simulink model "SLIPquadwalkold"  (R2015a)
settings: Solver=ode45  StartTime=0.0  StopTime=10  MaxStep=1e-3  RelTol=1e-4  AbsTol=1e-6
values from neighbouring files (symbols this model uses):
  blic = 0    [SLIPquad_paramswalk.m]    (also in purecmaeswalk.m; test.m)
  blx0 = x(10)    [SLIPquad_paramswalk.m]    (also in purecmaeswalk.m; test.m)
  bric = 1    [SLIPquad_paramswalk.m]    (also in purecmaeswalk.m; test.m)
  brx0 = 0    [SLIPquad_paramswalk.m]    (also in purecmaeswalk.m; test.m)
  flic = 0    [SLIPquad_paramswalk.m]    (also in purecmaeswalk.m; test.m)
  flx0 = x(9)    [SLIPquad_paramswalk.m]    (also in purecmaeswalk.m; test.m)
  fric = 1    [SLIPquad_paramswalk.m]    (also in purecmaeswalk.m; test.m)
  frx0 = 0    [SLIPquad_paramswalk.m]    (also in purecmaeswalk.m; test.m)
  g = 9.81    [SLIPquad_params - Copy.m]    (also in SLIPquad_params.m; SLIPquad_paramswalk.m; purecmaes.m; purecmaeswalk.m)
  J = 4.58    [SLIPquad_params - Copy.m]    (also in SLIPquad_params.m; SLIPquad_paramswalk.m; purecmaes.m; purecmaeswalk.m)
  L = 0.5    [SLIPquad_params - Copy.m]    (also in SLIPquad_params.m; SLIPquad_paramswalk.m; purecmaes.m; purecmaeswalk.m)
  l0 = 1    [SLIPquad_params - Copy.m]    (also in SLIPquad_params.m; SLIPquad_paramswalk.m; purecmaes.m; purecmaeswalk.m)
  m = 80    [SLIPquad_params - Copy.m]    (also in SLIPquad_params.m; SLIPquad_paramswalk.m; purecmaes.m; purecmaeswalk.m)
libraries: simulink_extras x4, dspswit3 x1
settings Model: Creator=hgeyer  LastModifiedBy=Joe
settings DataIOCC: LimitDataPoints=off  SignalLoggingSaveFormat=ModelDataLogs
settings OptimizationCC: ExpressionDepthLimit=2147483647
settings DebuggingCC: UnderspecifiedInitializationDetection=Classic  MergeDetectMultiDrivingBlocksExec=none  SolverPrmCheckMsg=warning  FcnCallInpInsideContextMsg=EnableAllAsWarning  StateNameClashWarn=warning

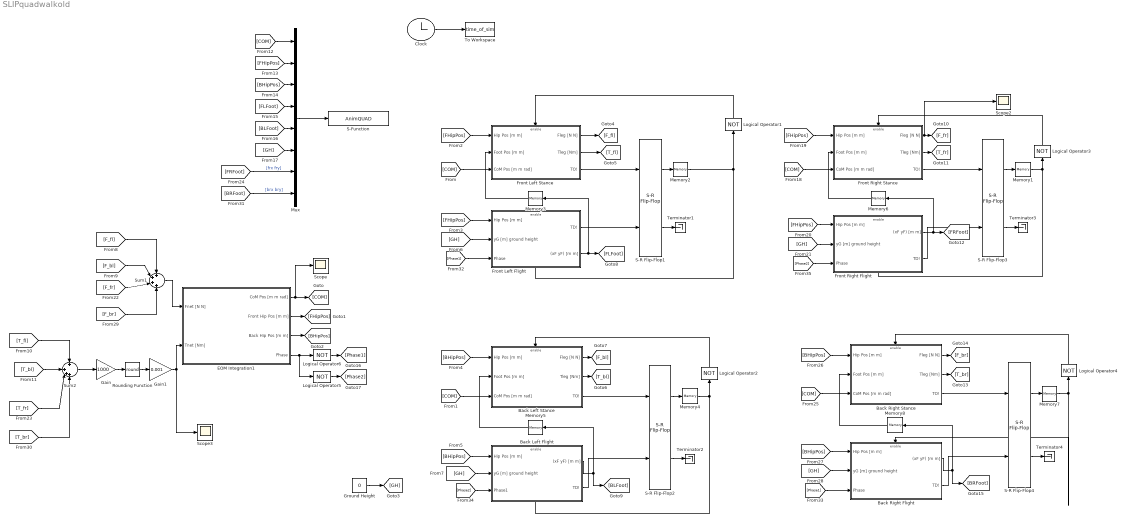
== system SLIPquadwalkold ==
  Back Left Flight : Subsystem
  Back Left Stance : Subsystem
  Back Right Flight : Subsystem
  Back Right Stance : Subsystem
  Clock : Clock
      settings: Decimation=100
  EOM Integration1 : Subsystem
  Front Left Flight : Subsystem
  Front Left Stance : Subsystem
  Front Right Flight : Subsystem
  Front Right Stance : Subsystem
  Gain : Gain  Gain=1000
  Gain1 : Gain  Gain=0.001
  Ground Height : Constant  Value=0
  Logical Operator{1..6} (6 alike) : Logic  Operator=NOT  AllPortsSameDT=off  OutDataTypeStr=boolean
  Memory1 : Memory  X0=fric
  Memory2 : Memory  X0=flic
  Memory3 : Memory  X0=[flx0 0]
  Memory4 : Memory  X0=blic
  Memory5 : Memory  X0=[blx0 0]
  Memory6 : Memory  X0=[frx0 0]
  Memory7 : Memory  X0=bric
  Memory8 : Memory  X0=[brx0 0]
  Mux : Mux  Inputs=8
  Rounding Function : Rounding  Operator=round
  S-Function : S-Function  FunctionName=AnimQUAD  Parameters=0.005  SFunctionDeploymentMode=off  EnableBusSupport=off
  S-R Flip-Flop1 : simulink_extras/Flip Flops/S-R Flip-Flop  initial_condition=flic
  S-R Flip-Flop2 : simulink_extras/Flip Flops/S-R Flip-Flop  initial_condition=blic
  S-R Flip-Flop3 : simulink_extras/Flip Flops/S-R Flip-Flop  initial_condition=fric
  S-R Flip-Flop4 : simulink_extras/Flip Flops/S-R Flip-Flop  initial_condition=bric
  Scope : Scope
      settings: TimeRange=auto  MaxDataPoints=5000  SaveToWorkspace=off  SaveName=ScopeData  YMin=-0.16878  YMax=0.96227  SampleTime=-1  DataFormat=Array
  Scope2 : Scope
      settings: TimeRange=auto  LimitDataPoints=on  MaxDataPoints=5000  SaveToWorkspace=off  SaveName=ScopeData3  YMin=-10  YMax=10  SampleTime=-1  DataFormat=Array
  Scope3 : Scope
      settings: TimeRange=auto  MaxDataPoints=5000  SaveToWorkspace=off  SaveName=ScopeData4  YMin=-0.05618  YMax=0.0173  SampleTime=-1  DataFormat=Array
  Sum1 : Sum  Inputs=++++
  Sum2 : Sum  Inputs=+|+++
  Terminator{1..4} (4 alike) : Terminator
  To Workspace : ToWorkspace  VariableName=time_of_sim  SampleTime=-1
      settings: MaxDataPoints=1
  wires:
  Front Left Stance/3(TO!) -> S-R Flip-Flop1/1
  S-R Flip-Flop1/1 -> Memory2/1
  Front Left Flight/1(TD!) -> S-R Flip-Flop1/2
  Logical Operator1/1 -> Front Left Stance/Enable
  S-R Flip-Flop1/2 -> Terminator1/1
  Front Left Flight/2((xF yF) [m m]) -> [FLFoot], Memory3/1
  Memory3/1 -> Front Left Stance/2(Foot Pos [m m])
  Back Left Stance/3(TO!) -> S-R Flip-Flop2/1
  S-R Flip-Flop2/1 -> Memory4/1
  Back Left Flight/2(TD!) -> S-R Flip-Flop2/2
  Memory4/1 -> Back Left Flight/Enable, Logical Operator2/1
  Logical Operator2/1 -> Back Left Stance/Enable
  S-R Flip-Flop2/2 -> Terminator2/1
  [GH] -> Back Left Flight/2(yG [m] ground height)
  Back Left Flight/1((xF yF) [m m]) -> [BLFoot], Memory5/1
  Memory5/1 -> Back Left Stance/2(Foot Pos [m m])
  Ground Height/1 -> [GH]
  [GH] -> Front Left Flight/2(yG [m] ground height)
  Front Left Stance/1(Fleg [N N]) -> [F_fl]
  Front Left Stance/2(Tleg [Nm]) -> [T_fl]
  Back Left Stance/1(Fleg [N N]) -> [F_bl]
  Back Left Stance/2(Tleg [Nm]) -> [T_bl]
  [F_fl] -> Sum1/1
  [F_bl] -> Sum1/2
  [T_fl] -> Sum2/1
  [T_bl] -> Sum2/2
  Sum1/1 -> EOM Integration1/1(Fnet [N N])
  EOM Integration1/1(CoM Pos [m m rad]) -> Scope/1, [COM]
  EOM Integration1/2(Front Hip Pos [m m]) -> [FHipPos]
  EOM Integration1/3(Back Hip Pos [m m]) -> [BHipPos]
  [FHipPos] -> Front Left Stance/1(Hip Pos [m m])
  [FHipPos] -> Front Left Flight/1(Hip Pos [m m])
  [BHipPos] -> Back Left Stance/1(Hip Pos [m m])
  [BHipPos] -> Back Left Flight/1(Hip Pos [m m])
  [COM] -> Front Left Stance/3(CoM Pos [m m rad])
  [COM] -> Back Left Stance/3(CoM Pos [m m rad])
  Sum2/1 -> Gain/1
  Gain1/1 -> Scope3/1, EOM Integration1/2(Tnet [Nm])
  Gain/1 -> Rounding Function/1
  Rounding Function/1 -> Gain1/1
  Mux/1 -> S-Function/1
  [COM] -> Mux/1
  [FHipPos] -> Mux/2
  [BHipPos] -> Mux/3
  [FLFoot] -> Mux/4
  [BLFoot] -> Mux/5
  [GH] -> Mux/6
  [FRFoot] -> Mux/7  "[frx fry]"
  [BRFoot] -> Mux/8  "[brx bry]"
  Front Right Stance/3(TO!) -> S-R Flip-Flop3/1
  S-R Flip-Flop3/1 -> Memory1/1
  Front Right Flight/2(TD!) -> S-R Flip-Flop3/2
  Memory1/1 -> Front Right Flight/Enable, Logical Operator3/1
  Logical Operator3/1 -> Front Right Stance/Enable
  S-R Flip-Flop3/2 -> Terminator3/1
  Front Right Flight/1((xF yF) [m m]) -> Memory6/1, [FRFoot]
  Memory6/1 -> Front Right Stance/2(Foot Pos [m m])
  [GH] -> Front Right Flight/2(yG [m] ground height)
  Front Right Stance/1(Fleg [N N]) -> Scope2/1, [F_fr]
  Front Right Stance/2(Tleg [Nm]) -> [T_fr]
  [FHipPos] -> Front Right Stance/1(Hip Pos [m m])
  [FHipPos] -> Front Right Flight/1(Hip Pos [m m])
  [COM] -> Front Right Stance/3(CoM Pos [m m rad])
  [F_fr] -> Sum1/3
  [T_fr] -> Sum2/3
  Back Right Stance/3(TO!) -> S-R Flip-Flop4/1
  S-R Flip-Flop4/1 -> Memory7/1
  Back Right Flight/2(TD!) -> S-R Flip-Flop4/2
  Memory7/1 -> Back Right Flight/Enable, Logical Operator4/1
  Logical Operator4/1 -> Back Right Stance/Enable
  S-R Flip-Flop4/2 -> Terminator4/1
  [GH] -> Back Right Flight/2(yG [m] ground height)
  Back Right Flight/1((xF yF) [m m]) -> [BRFoot], Memory8/1
  Memory8/1 -> Back Right Stance/2(Foot Pos [m m])
  Back Right Stance/1(Fleg [N N]) -> [F_br]
  Back Right Stance/2(Tleg [Nm]) -> [T_br]
  [BHipPos] -> Back Right Stance/1(Hip Pos [m m])
  [BHipPos] -> Back Right Flight/1(Hip Pos [m m])
  [COM] -> Back Right Stance/3(CoM Pos [m m rad])
  [F_br] -> Sum1/4
  [T_br] -> Sum2/4
  Clock/1 -> To Workspace/1
  EOM Integration1/4(Phase) -> Logical Operator5/1, Logical Operator6/1
  [Phase1] -> Front Left Flight/3(Phase)
  [Phase1] -> Back Right Flight/3(Phase)
  [Phase2] -> Back Left Flight/3(Phase1)
  [Phase2] -> Front Right Flight/3(Phase)
  Logical Operator5/1 -> [Phase2]
  Logical Operator6/1 -> [Phase1]
  Memory2/1 -> Front Left Flight/Enable, Logical Operator1/1

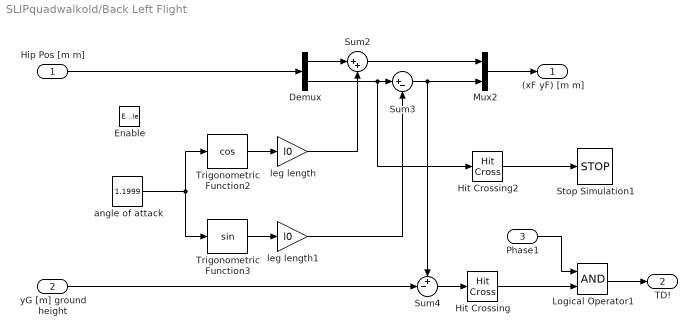
== system SLIPquadwalkold/Back Left Flight ==
  Hip Pos [m m] : Inport
  yG [m] ground height : Inport  Port=2
  Phase1 : Inport  Port=3
  Enable : EnablePort  StatesWhenEnabling=reset
  Demux : Demux  Outputs=2
  Hit Crossing : HitCross  HitCrossingDirection=falling
  Hit Crossing2 : HitCross  HitCrossingOffset=-1  HitCrossingDirection=falling
  Logical Operator1 : Logic  AllPortsSameDT=off  OutDataTypeStr=boolean
  Mux2 : Mux  Inputs=2
  Stop Simulation1 : Stop
  Sum2 : Sum  Inputs=|++
  Sum3 : Sum  Inputs=|+-
  Sum4 : Sum  Inputs=+-|
  Trigonometric Function2 : Trigonometry  Operator=cos
  Trigonometric Function3 : Trigonometry
  angle of attack : Constant  Value=1.1999
  leg length : Gain  Gain=l0
  leg length1 : Gain  Gain=l0
  (xF yF) [m m] : Outport  InitialOutput=[blx0 0]
      settings: AttributesFormatString=%<OutputWhenDisabled>
  TD! : Outport  Port=2  OutputWhenDisabled=reset  InitialOutput=0
      settings: AttributesFormatString=%<OutputWhenDisabled>
  wires:
  Demux/2 -> Hit Crossing2/1, Sum3/1
  Demux/1 -> Sum2/1
  angle of attack/1 -> Trigonometric Function3/1, Trigonometric Function2/1
  Trigonometric Function2/1 -> leg length/1
  Trigonometric Function3/1 -> leg length1/1
  Hip Pos [m m]/1 -> Demux/1
  leg length/1 -> Sum2/2
  leg length1/1 -> Sum3/2
  Sum3/1 -> Mux2/2, Sum4/1
  Sum2/1 -> Mux2/1
  Mux2/1 -> (xF yF) [m m]/1
  yG [m] ground height/1 -> Sum4/2
  Sum4/1 -> Hit Crossing/1
  Hit Crossing2/1 -> Stop Simulation1/1
  Hit Crossing/1 -> Logical Operator1/2
  Phase1/1 -> Logical Operator1/1
  Logical Operator1/1 -> TD!/1

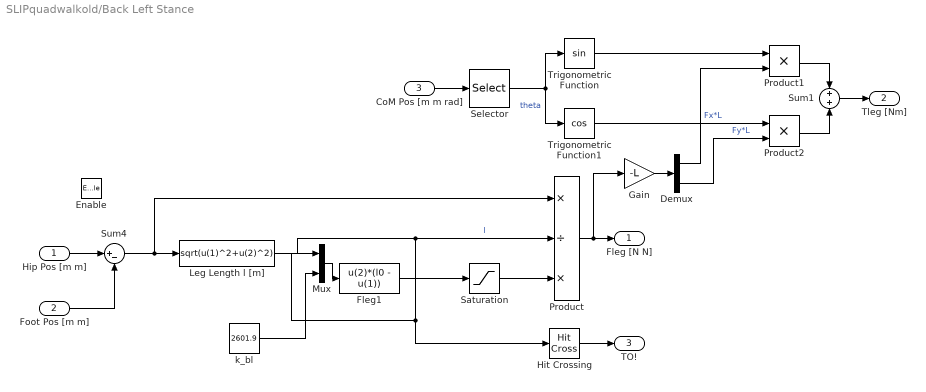
== system SLIPquadwalkold/Back Left Stance ==
  Hip Pos [m m] : Inport
  Foot Pos [m m] : Inport  Port=2
  CoM Pos [m m rad] : Inport  Port=3
  Enable : EnablePort  StatesWhenEnabling=reset
  Demux : Demux  Outputs=2
  Fleg1 : Fcn  Expr=u(2)*(l0 - u(1))
  Gain : Gain  Gain=-L
  Hit Crossing : HitCross  HitCrossingOffset=l0  HitCrossingDirection=rising
  Leg Length l [m] : Fcn  Expr=sqrt(u(1)^2+u(2)^2)
  Mux : Mux  Inputs=2
  Product : Product  Inputs=*/*
  Product1 : Product
  Product2 : Product
  Saturation : Saturate  UpperLimit=Inf  LowerLimit=0
  Selector : Selector  InputPortWidth=3  IndexOptions=Index vector (dialog)  Indices=[3]  OutputSizes=1
  Sum1 : Sum  Inputs=+|+
  Sum4 : Sum  Inputs=|+-
  Trigonometric Function : Trigonometry
  Trigonometric Function1 : Trigonometry  Operator=cos
  k_bl : Constant  Value=2601.9
  Fleg [N N] : Outport  OutputWhenDisabled=reset  InitialOutput=[0 0]
      settings: AttributesFormatString=%<OutputWhenDisabled>
  Tleg [Nm] : Outport  Port=2  OutputWhenDisabled=reset  InitialOutput=[0]
      settings: AttributesFormatString=%<OutputWhenDisabled>
  TO! : Outport  Port=3  OutputWhenDisabled=reset  InitialOutput=[0]
      settings: AttributesFormatString=%<OutputWhenDisabled>
  wires:
  Sum1/1 -> Tleg [Nm]/1
  Product1/1 -> Sum1/1
  Product2/1 -> Sum1/2
  Gain/1 -> Demux/1
  Demux/2 -> Product2/2  "Fy*L"
  Demux/1 -> Product1/2  "Fx*L"
  Trigonometric Function/1 -> Product1/1
  Trigonometric Function1/1 -> Product2/1
  Selector/1 -> Trigonometric Function/1, Trigonometric Function1/1  "theta"
  CoM Pos [m m rad]/1 -> Selector/1
  Foot Pos [m m]/1 -> Sum4/2
  Hip Pos [m m]/1 -> Sum4/1
  Hit Crossing/1 -> TO!/1
  Product/1 -> Fleg [N N]/1, Gain/1
  Fleg1/1 -> Saturation/1
  Leg Length l [m]/1 -> Hit Crossing/1, Mux/1, Product/2  "l"
  Sum4/1 -> Leg Length l [m]/1, Product/1
  Mux/1 -> Fleg1/1
  k_bl/1 -> Mux/2
  Saturation/1 -> Product/3

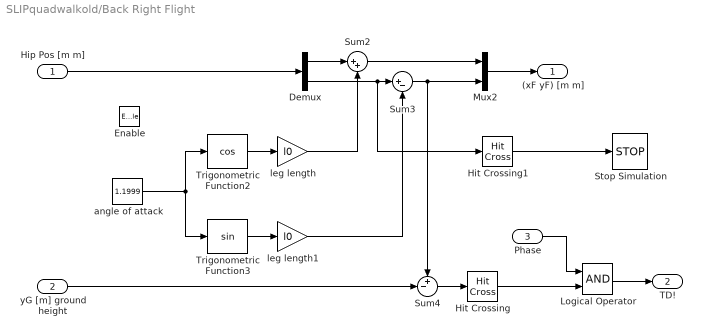
== system SLIPquadwalkold/Back Right Flight ==
  Hip Pos [m m] : Inport
  yG [m] ground height : Inport  Port=2
  Phase : Inport  Port=3
  Enable : EnablePort  StatesWhenEnabling=reset
  Demux : Demux  Outputs=2
  Hit Crossing : HitCross  HitCrossingDirection=falling
  Hit Crossing1 : HitCross  HitCrossingOffset=-1  HitCrossingDirection=falling
  Logical Operator : Logic  AllPortsSameDT=off  OutDataTypeStr=boolean
  Mux2 : Mux  Inputs=2
  Stop Simulation : Stop
  Sum2 : Sum  Inputs=|++
  Sum3 : Sum  Inputs=|+-
  Sum4 : Sum  Inputs=+-|
  Trigonometric Function2 : Trigonometry  Operator=cos
  Trigonometric Function3 : Trigonometry
  angle of attack : Constant  Value=1.1999
  leg length : Gain  Gain=l0
  leg length1 : Gain  Gain=l0
  (xF yF) [m m] : Outport  InitialOutput=[brx0 0]
      settings: AttributesFormatString=%<OutputWhenDisabled>
  TD! : Outport  Port=2  OutputWhenDisabled=reset  InitialOutput=0
      settings: AttributesFormatString=%<OutputWhenDisabled>
  wires:
  Demux/2 -> Hit Crossing1/1, Sum3/1
  Demux/1 -> Sum2/1
  angle of attack/1 -> Trigonometric Function3/1, Trigonometric Function2/1
  Trigonometric Function2/1 -> leg length/1
  Trigonometric Function3/1 -> leg length1/1
  Hip Pos [m m]/1 -> Demux/1
  leg length/1 -> Sum2/2
  leg length1/1 -> Sum3/2
  Sum3/1 -> Mux2/2, Sum4/1
  Sum2/1 -> Mux2/1
  Mux2/1 -> (xF yF) [m m]/1
  yG [m] ground height/1 -> Sum4/2
  Sum4/1 -> Hit Crossing/1
  Hit Crossing1/1 -> Stop Simulation/1
  Hit Crossing/1 -> Logical Operator/2
  Phase/1 -> Logical Operator/1
  Logical Operator/1 -> TD!/1

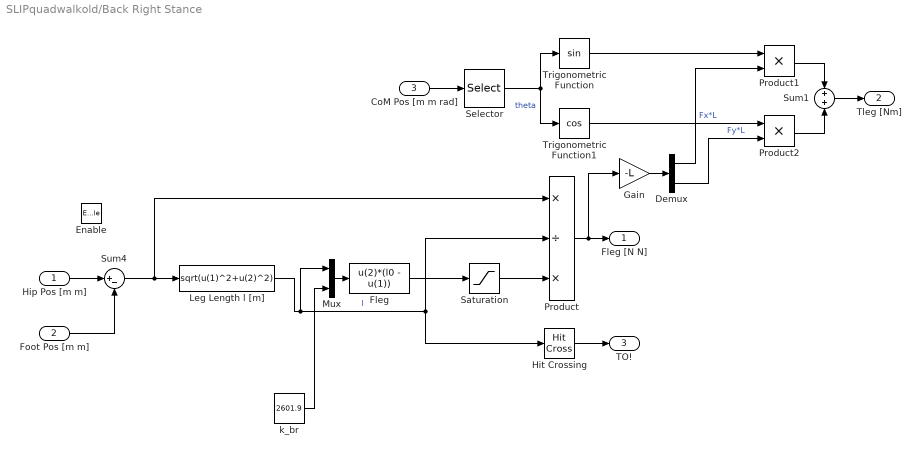
== system SLIPquadwalkold/Back Right Stance ==
  Hip Pos [m m] : Inport
  Foot Pos [m m] : Inport  Port=2
  CoM Pos [m m rad] : Inport  Port=3
  Enable : EnablePort  StatesWhenEnabling=reset
  Demux : Demux  Outputs=2
  Fleg : Fcn  Expr=u(2)*(l0 - u(1))
  Gain : Gain  Gain=-L
  Hit Crossing : HitCross  HitCrossingOffset=l0  HitCrossingDirection=rising
  Leg Length l [m] : Fcn  Expr=sqrt(u(1)^2+u(2)^2)
  Mux : Mux  Inputs=2
  Product : Product  Inputs=*/*
  Product1 : Product
  Product2 : Product
  Saturation : Saturate  UpperLimit=Inf  LowerLimit=0
  Selector : Selector  InputPortWidth=3  IndexOptions=Index vector (dialog)  Indices=[3]  OutputSizes=1
  Sum1 : Sum  Inputs=+|+
  Sum4 : Sum  Inputs=|+-
  Trigonometric Function : Trigonometry
  Trigonometric Function1 : Trigonometry  Operator=cos
  k_br : Constant  Value=2601.9
  Fleg [N N] : Outport  OutputWhenDisabled=reset  InitialOutput=[0 0]
      settings: AttributesFormatString=%<OutputWhenDisabled>
  Tleg [Nm] : Outport  Port=2  OutputWhenDisabled=reset  InitialOutput=[0]
      settings: AttributesFormatString=%<OutputWhenDisabled>
  TO! : Outport  Port=3  OutputWhenDisabled=reset  InitialOutput=[0]
      settings: AttributesFormatString=%<OutputWhenDisabled>
  wires:
  Sum1/1 -> Tleg [Nm]/1
  Product1/1 -> Sum1/1
  Product2/1 -> Sum1/2
  Gain/1 -> Demux/1
  Demux/2 -> Product2/2  "Fy*L"
  Demux/1 -> Product1/2  "Fx*L"
  Trigonometric Function/1 -> Product1/1
  Trigonometric Function1/1 -> Product2/1
  Selector/1 -> Trigonometric Function/1, Trigonometric Function1/1  "theta"
  CoM Pos [m m rad]/1 -> Selector/1
  Foot Pos [m m]/1 -> Sum4/2
  Hip Pos [m m]/1 -> Sum4/1
  Hit Crossing/1 -> TO!/1
  Product/1 -> Fleg [N N]/1, Gain/1
  Fleg/1 -> Saturation/1
  Leg Length l [m]/1 -> Hit Crossing/1, Product/2, Mux/1  "l"
  Sum4/1 -> Leg Length l [m]/1, Product/1
  Mux/1 -> Fleg/1
  k_br/1 -> Mux/2
  Saturation/1 -> Product/3

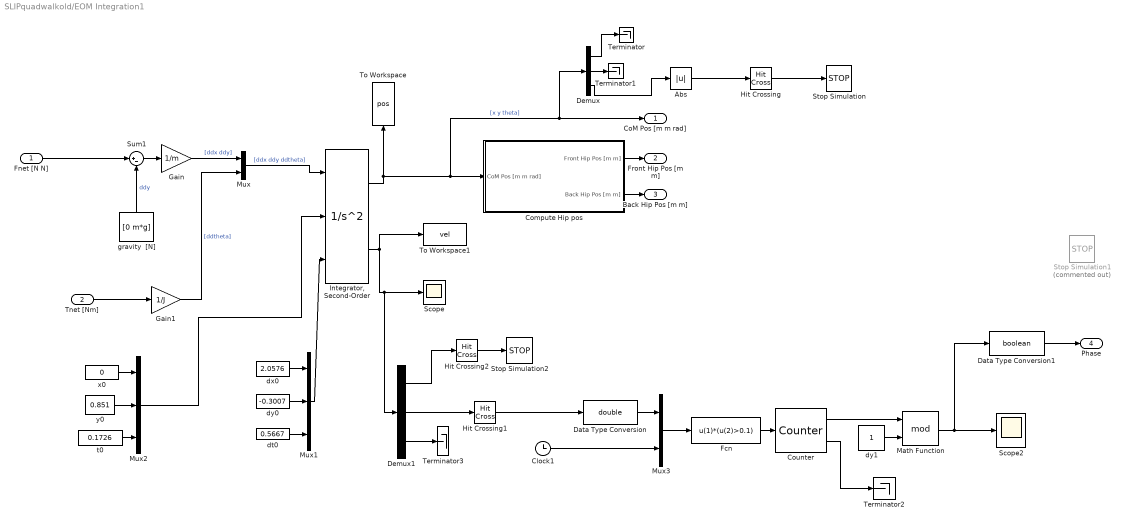
== system SLIPquadwalkold/EOM Integration1 ==
  Fnet [N N] : Inport
  Tnet [Nm] : Inport  Port=2
  Abs : Abs
  Clock1 : Clock
  Compute Hip pos : Subsystem
  Counter : dspswit3/Counter  Direction=Up  CountEvent=Rising edge  CounterSize=User defined  MaxCount=100000  InitialCount=0  Output=Count and Hit  HitValue=32  ResetInput=off  SamplesPerFrame=1  Ts=1  CntDtype=double  HitDtype=Logical
  Data Type Conversion : DataTypeConversion  OutDataTypeStr=double
  Data Type Conversion1 : DataTypeConversion  OutDataTypeStr=boolean
  Demux : Demux  Outputs=3
  Demux1 : Demux  Outputs=3
  Fcn : Fcn  Expr=u(1)*(u(2)>0.1)
  Gain : Gain  Gain=1/m
  Gain1 : Gain  Gain=1/J
  Hit Crossing : HitCross  HitCrossingOffset=1.57
  Hit Crossing1 : HitCross  HitCrossingOffset=0.0001  HitCrossingDirection=falling
  Hit Crossing2 : HitCross  HitCrossingDirection=falling
  "Integrator, Second-Order" : SecondOrderIntegrator  ICSourceX=external  ICSourceDXDT=external
  Math Function : Math  Operator=mod  SaturateOnIntegerOverflow=on
  Mux : Mux  Inputs=2
  Mux1 : Mux  Inputs=3
  Mux2 : Mux  Inputs=3
  Mux3 : Mux  Inputs=2
  Scope : Scope
      settings: TimeRange=3.298211913921595  MaxDataPoints=5000  SaveToWorkspace=off  SaveName=ScopeData2  YMin=-10  YMax=10  SampleTime=-1  DataFormat=Array
  Scope2 : Scope
      settings: TimeRange=auto  MaxDataPoints=5000  SaveToWorkspace=off  SaveName=ScopeData2  YMin=-0.25  YMax=2.25  SampleTime=-1
  Stop Simulation : Stop
  Stop Simulation1 : Stop  Commented=on
  Stop Simulation2 : Stop
  Sum1 : Sum  Inputs=|+-
  Terminator{,1..3} (4 alike) : Terminator
  To Workspace : ToWorkspace  VariableName=pos  SampleTime=-1
  To Workspace1 : ToWorkspace  VariableName=vel  SampleTime=-1
  dt0 : Constant  Value=0.5667
  dx0 : Constant  Value=2.0576
  dy0 : Constant  Value=-0.3007
  dy1 : Constant
  gravity  [N] : Constant  Value=[0 m*g]
  t0 : Constant  Value=0.1726
  x0 : Constant  Value=0
  y0 : Constant  Value=0.851
  CoM Pos [m m rad] : Outport
  Front Hip Pos [m m] : Outport  Port=2
  Back Hip Pos [m m] : Outport  Port=3
  Phase : Outport  Port=4
  wires:
  Compute Hip pos/1(Front Hip Pos [m m]) -> Front Hip Pos [m m]/1
  "Integrator, Second-Order"/1 -> To Workspace/1, Demux/1, CoM Pos [m m rad]/1, Compute Hip pos/1(CoM Pos [m m rad])  "[x y theta]"
  Tnet [Nm]/1 -> Gain1/1
  Gain1/1 -> Mux/2  "[ddtheta]"
  Mux/1 -> "Integrator, Second-Order"/1  "[ddx ddy ddtheta]"
  Fnet [N N]/1 -> Sum1/1
  Gain/1 -> Mux/1  "[ddx ddy]"
  Mux2/1 -> "Integrator, Second-Order"/2
  gravity  [N]/1 -> Sum1/2  "ddy"
  Sum1/1 -> Gain/1
  Compute Hip pos/2(Back Hip Pos [m m]) -> Back Hip Pos [m m]/1
  Mux1/1 -> "Integrator, Second-Order"/3
  dx0/1 -> Mux1/1
  dy0/1 -> Mux1/2
  dt0/1 -> Mux1/3
  Demux/3 -> Abs/1
  Demux/1 -> Terminator/1
  Demux/2 -> Terminator1/1
  Hit Crossing/1 -> Stop Simulation/1
  Abs/1 -> Hit Crossing/1
  Hit Crossing1/1 -> Data Type Conversion/1
  "Integrator, Second-Order"/2 -> To Workspace1/1, Demux1/1, Scope/1
  Demux1/3 -> Terminator3/1
  x0/1 -> Mux2/1
  y0/1 -> Mux2/2
  t0/1 -> Mux2/3
  Demux1/2 -> Hit Crossing1/1
  Demux1/1 -> Hit Crossing2/1
  Clock1/1 -> Mux3/2
  Mux3/1 -> Fcn/1
  Data Type Conversion/1 -> Mux3/1
  Fcn/1 -> Counter/1
  Counter/1 -> Math Function/1
  dy1/1 -> Math Function/2
  Math Function/1 -> Scope2/1, Data Type Conversion1/1
  Data Type Conversion1/1 -> Phase/1
  Hit Crossing2/1 -> Stop Simulation2/1
  Counter/2 -> Terminator2/1

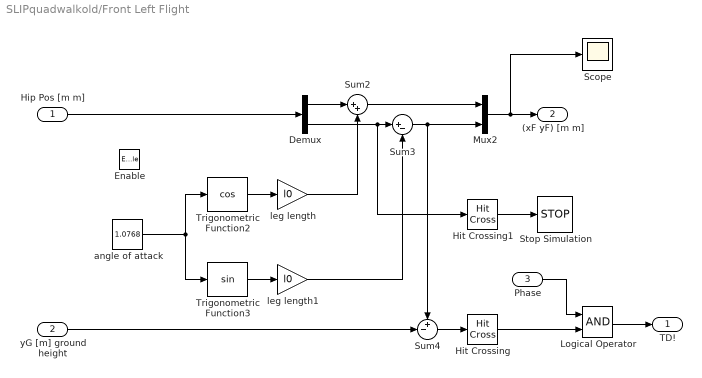
== system SLIPquadwalkold/Front Left Flight ==
  Hip Pos [m m] : Inport
  yG [m] ground height : Inport  Port=2
  Phase : Inport  Port=3
  Enable : EnablePort  StatesWhenEnabling=reset
  Demux : Demux  Outputs=2
  Hit Crossing : HitCross  HitCrossingDirection=falling
  Hit Crossing1 : HitCross  HitCrossingOffset=-1  HitCrossingDirection=falling
  Logical Operator : Logic  AllPortsSameDT=off  OutDataTypeStr=boolean
  Mux2 : Mux  Inputs=2
  Scope : Scope
      settings: TimeRange=auto  MaxDataPoints=5000  SaveToWorkspace=off  YMin=-0.08015  YMax=1.67767  SampleTime=-1
  Stop Simulation : Stop
  Sum2 : Sum  Inputs=|++
  Sum3 : Sum  Inputs=|+-
  Sum4 : Sum  Inputs=+-|
  Trigonometric Function2 : Trigonometry  Operator=cos
  Trigonometric Function3 : Trigonometry
  angle of attack : Constant  Value=1.0768
  leg length : Gain  Gain=l0
  leg length1 : Gain  Gain=l0
  TD! : Outport  OutputWhenDisabled=reset  InitialOutput=0
      settings: AttributesFormatString=%<OutputWhenDisabled>
  (xF yF) [m m] : Outport  Port=2  InitialOutput=[flx0 0]
      settings: AttributesFormatString=%<OutputWhenDisabled>
  wires:
  Hit Crossing1/1 -> Stop Simulation/1
  Sum4/1 -> Hit Crossing/1
  yG [m] ground height/1 -> Sum4/2
  Mux2/1 -> Scope/1, (xF yF) [m m]/1
  Sum2/1 -> Mux2/1
  Sum3/1 -> Sum4/1, Mux2/2
  leg length1/1 -> Sum3/2
  leg length/1 -> Sum2/2
  Hip Pos [m m]/1 -> Demux/1
  Trigonometric Function3/1 -> leg length1/1
  Trigonometric Function2/1 -> leg length/1
  angle of attack/1 -> Trigonometric Function2/1, Trigonometric Function3/1
  Demux/1 -> Sum2/1
  Demux/2 -> Sum3/1, Hit Crossing1/1
  Hit Crossing/1 -> Logical Operator/2
  Phase/1 -> Logical Operator/1
  Logical Operator/1 -> TD!/1

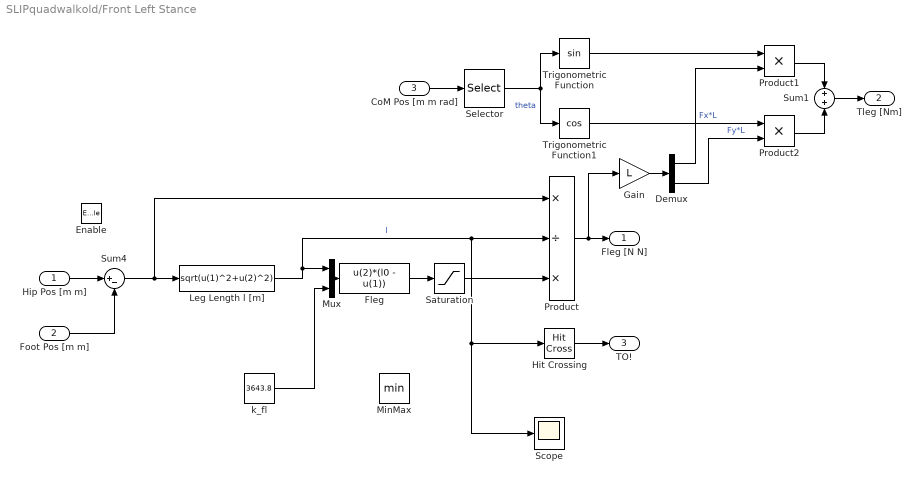
== system SLIPquadwalkold/Front Left Stance ==
  Hip Pos [m m] : Inport
  Foot Pos [m m] : Inport  Port=2
  CoM Pos [m m rad] : Inport  Port=3
  Enable : EnablePort  StatesWhenEnabling=reset
  Demux : Demux  Outputs=2
  Fleg : Fcn  Expr=u(2)*(l0 - u(1))
  Gain : Gain  Gain=L
  Hit Crossing : HitCross  HitCrossingOffset=l0  HitCrossingDirection=rising
  Leg Length l [m] : Fcn  Expr=sqrt(u(1)^2+u(2)^2)
  MinMax : MinMax
  Mux : Mux  Inputs=2
  Product : Product  Inputs=*/*
  Product1 : Product
  Product2 : Product
  Saturation : Saturate  UpperLimit=Inf  LowerLimit=0
  Scope : Scope
      settings: TimeRange=auto  MaxDataPoints=5000  SaveToWorkspace=off  SaveName=ScopeData4  YMin=0.51566  YMax=3.15238  SampleTime=-1
  Selector : Selector  InputPortWidth=3  IndexOptions=Index vector (dialog)  Indices=[3]  OutputSizes=1
  Sum1 : Sum  Inputs=+|+
  Sum4 : Sum  Inputs=|+-
  Trigonometric Function : Trigonometry
  Trigonometric Function1 : Trigonometry  Operator=cos
  k_fl : Constant  Value=3643.8
  Fleg [N N] : Outport  OutputWhenDisabled=reset  InitialOutput=[0 0]
      settings: AttributesFormatString=%<OutputWhenDisabled>
  Tleg [Nm] : Outport  Port=2  OutputWhenDisabled=reset  InitialOutput=[0]
      settings: AttributesFormatString=%<OutputWhenDisabled>
  TO! : Outport  Port=3  OutputWhenDisabled=reset  InitialOutput=[0]
      settings: AttributesFormatString=%<OutputWhenDisabled>
  wires:
  Sum4/1 -> Product/1, Leg Length l [m]/1
  Leg Length l [m]/1 -> Mux/1, Hit Crossing/1, Scope/1, Product/2  "l"
  Fleg/1 -> Saturation/1
  Product/1 -> Gain/1, Fleg [N N]/1
  Hit Crossing/1 -> TO!/1
  Hip Pos [m m]/1 -> Sum4/1
  Foot Pos [m m]/1 -> Sum4/2
  CoM Pos [m m rad]/1 -> Selector/1
  Selector/1 -> Trigonometric Function1/1, Trigonometric Function/1  "theta"
  Trigonometric Function1/1 -> Product2/1
  Trigonometric Function/1 -> Product1/1
  Demux/1 -> Product1/2  "Fx*L"
  Demux/2 -> Product2/2  "Fy*L"
  Gain/1 -> Demux/1
  Product2/1 -> Sum1/2
  Product1/1 -> Sum1/1
  Sum1/1 -> Tleg [Nm]/1
  Mux/1 -> Fleg/1
  k_fl/1 -> Mux/2
  Saturation/1 -> Product/3

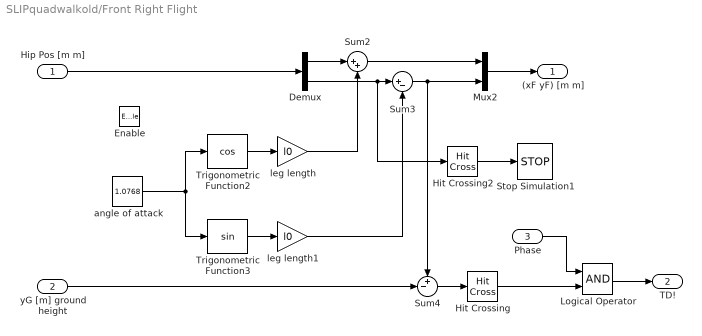
== system SLIPquadwalkold/Front Right Flight ==
  Hip Pos [m m] : Inport
  yG [m] ground height : Inport  Port=2
  Phase : Inport  Port=3
  Enable : EnablePort  StatesWhenEnabling=reset
  Demux : Demux  Outputs=2
  Hit Crossing : HitCross  HitCrossingDirection=falling
  Hit Crossing2 : HitCross  HitCrossingOffset=-1  HitCrossingDirection=falling
  Logical Operator : Logic  AllPortsSameDT=off  OutDataTypeStr=boolean
  Mux2 : Mux  Inputs=2
  Stop Simulation1 : Stop
  Sum2 : Sum  Inputs=|++
  Sum3 : Sum  Inputs=|+-
  Sum4 : Sum  Inputs=+-|
  Trigonometric Function2 : Trigonometry  Operator=cos
  Trigonometric Function3 : Trigonometry
  angle of attack : Constant  Value=1.0768
  leg length : Gain  Gain=l0
  leg length1 : Gain  Gain=l0
  (xF yF) [m m] : Outport  InitialOutput=[frx0 0]
      settings: AttributesFormatString=%<OutputWhenDisabled>
  TD! : Outport  Port=2  OutputWhenDisabled=reset  InitialOutput=0
      settings: AttributesFormatString=%<OutputWhenDisabled>
  wires:
  Sum4/1 -> Hit Crossing/1
  yG [m] ground height/1 -> Sum4/2
  Mux2/1 -> (xF yF) [m m]/1
  Sum2/1 -> Mux2/1
  Sum3/1 -> Sum4/1, Mux2/2
  leg length1/1 -> Sum3/2
  leg length/1 -> Sum2/2
  Hip Pos [m m]/1 -> Demux/1
  Trigonometric Function3/1 -> leg length1/1
  Trigonometric Function2/1 -> leg length/1
  angle of attack/1 -> Trigonometric Function2/1, Trigonometric Function3/1
  Demux/1 -> Sum2/1
  Demux/2 -> Hit Crossing2/1, Sum3/1
  Hit Crossing2/1 -> Stop Simulation1/1
  Hit Crossing/1 -> Logical Operator/2
  Phase/1 -> Logical Operator/1
  Logical Operator/1 -> TD!/1

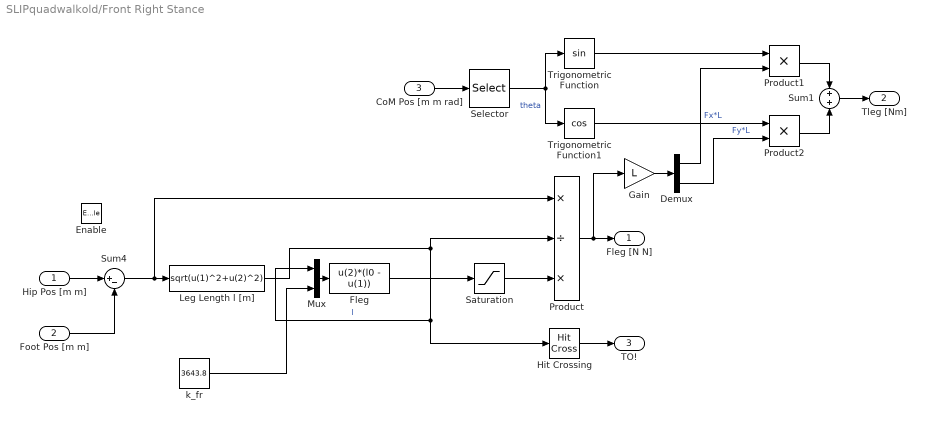
== system SLIPquadwalkold/Front Right Stance ==
  Hip Pos [m m] : Inport
  Foot Pos [m m] : Inport  Port=2
  CoM Pos [m m rad] : Inport  Port=3
  Enable : EnablePort  StatesWhenEnabling=reset
  Demux : Demux  Outputs=2
  Fleg : Fcn  Expr=u(2)*(l0 - u(1))
  Gain : Gain  Gain=L
  Hit Crossing : HitCross  HitCrossingOffset=l0  HitCrossingDirection=rising
  Leg Length l [m] : Fcn  Expr=sqrt(u(1)^2+u(2)^2)
  Mux : Mux  Inputs=2
  Product : Product  Inputs=*/*
  Product1 : Product
  Product2 : Product
  Saturation : Saturate  UpperLimit=Inf  LowerLimit=0
  Selector : Selector  InputPortWidth=3  IndexOptions=Index vector (dialog)  Indices=[3]  OutputSizes=1
  Sum1 : Sum  Inputs=+|+
  Sum4 : Sum  Inputs=|+-
  Trigonometric Function : Trigonometry
  Trigonometric Function1 : Trigonometry  Operator=cos
  k_fr : Constant  Value=3643.8
  Fleg [N N] : Outport  OutputWhenDisabled=reset  InitialOutput=[0 0]
      settings: AttributesFormatString=%<OutputWhenDisabled>
  Tleg [Nm] : Outport  Port=2  OutputWhenDisabled=reset  InitialOutput=[0]
      settings: AttributesFormatString=%<OutputWhenDisabled>
  TO! : Outport  Port=3  OutputWhenDisabled=reset  InitialOutput=[0]
      settings: AttributesFormatString=%<OutputWhenDisabled>
  wires:
  Sum4/1 -> Product/1, Leg Length l [m]/1
  Leg Length l [m]/1 -> Mux/1, Hit Crossing/1, Product/2  "l"
  Fleg/1 -> Saturation/1
  Product/1 -> Gain/1, Fleg [N N]/1
  Hit Crossing/1 -> TO!/1
  Hip Pos [m m]/1 -> Sum4/1
  Foot Pos [m m]/1 -> Sum4/2
  CoM Pos [m m rad]/1 -> Selector/1
  Selector/1 -> Trigonometric Function1/1, Trigonometric Function/1  "theta"
  Trigonometric Function1/1 -> Product2/1
  Trigonometric Function/1 -> Product1/1
  Demux/1 -> Product1/2  "Fx*L"
  Demux/2 -> Product2/2  "Fy*L"
  Gain/1 -> Demux/1
  Product2/1 -> Sum1/2
  Product1/1 -> Sum1/1
  Sum1/1 -> Tleg [Nm]/1
  Mux/1 -> Fleg/1
  k_fr/1 -> Mux/2
  Saturation/1 -> Product/3

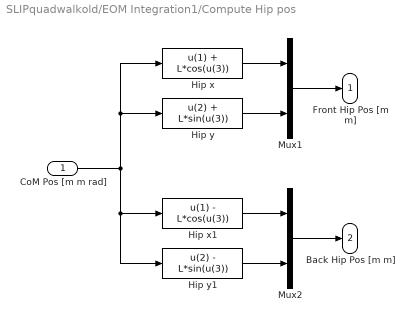
== system SLIPquadwalkold/EOM Integration1/Compute Hip pos ==
  CoM Pos [m m rad] : Inport
  Hip x : Fcn  Expr=u(1) + L*cos(u(3))
  Hip x1 : Fcn  Expr=u(1) - L*cos(u(3))
  Hip y : Fcn  Expr=u(2) + L*sin(u(3))
  Hip y1 : Fcn  Expr=u(2) - L*sin(u(3))
  Mux1 : Mux  Inputs=2
  Mux2 : Mux  Inputs=2
  Front Hip Pos [m m] : Outport
  Back Hip Pos [m m] : Outport  Port=2
  wires:
  Hip y/1 -> Mux1/2
  Mux1/1 -> Front Hip Pos [m m]/1
  Hip x/1 -> Mux1/1
  Hip y1/1 -> Mux2/2
  Mux2/1 -> Back Hip Pos [m m]/1
  Hip x1/1 -> Mux2/1
  CoM Pos [m m rad]/1 -> Hip x/1, Hip y/1, Hip y1/1, Hip x1/1
